simulink model "EngBrk_ExhFlpCtl"  (R2016b)
settings: configuration reference "CodeGenConfigSet" (kept outside this file)
values from neighbouring files (symbols this model uses):
  EngBrk_pExhFlpBstDflVal_C = Calibration.Parameter    [init_EngBrk_ExhFlpCtl.m]
  EngBrk_pExhFlpBstOn_C = Calibration.Parameter    [init_EngBrk_ExhFlpCtl.m]
  EngBrk_rExhFlpBrkLvl_C = Calibration.Parameter    [init_EngBrk_ExhFlpCtl.m]
  EngBrk_tiExhFlpBstOn_C = Calibration.Parameter    [init_EngBrk_ExhFlpCtl.m]
  PRC_ZERO = uint8(0)    [init_EngBrk_ExhFlpCtl.m]
undefined symbols (not defined in the file or in its folder): EngBrk_ExhFlpCtl_DT
settings Model: Creator=lenovo  LastModifiedBy=lenovo
settings ConfigSetRef: SourceLocation=Base Workspace

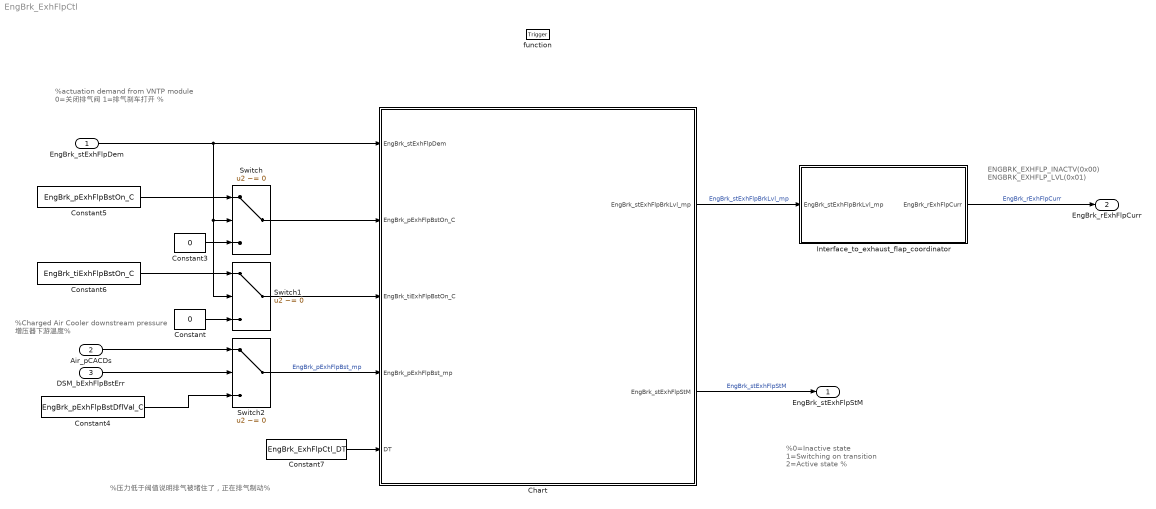
== system EngBrk_ExhFlpCtl ==
  note: %actuation demand from VNTP module
      | 0=关闭排气阀
      | 1=排气刹车打开 %
  note: ENGBRK_EXHFLP_INACTV(0x00)
      | ENGBRK_EXHFLP_LVL(0x01)
  note: %0=Inactive state
      | 1=Switching on transition
      | 2=Active state %
  note: %Charged Air Cooler downstream pressure
      | 增压器下游温度%
  note: %压力低于阀值说明排气被堵住了，正在排气制动%
  EngBrk_stExhFlpDem : Inport  Description=Activation demand to exhaust flap  OutMin=0  OutMax=1  OutDataTypeStr=boolean
  Air_pCACDs : Inport  Tag=kPa  Description=Air pressure downstream of the charge air cooler  Port=2  OutMin=-3276.8  OutMax=3276.7  OutDataTypeStr=AirPressure_kPa
  DSM_bExhFlpBstErr : Inport  Description=state of FId_ExhFlpBstErr  Port=3  OutMin=0  OutMax=1  OutDataTypeStr=boolean
  function : TriggerPort  TriggerType=function-call  VariantControl=Variant
  Chart : Stateflow chart  TreatAsAtomicUnit=on
  Constant : Constant  Value=0  OutDataTypeStr=Inherit: Inherit via back propagation
  Constant3 : Constant  Value=0  OutDataTypeStr=Inherit: Inherit via back propagation
  Constant4 : Constant  Value=EngBrk_pExhFlpBstDflVal_C
  Constant5 : Constant  Value=EngBrk_pExhFlpBstOn_C
  Constant6 : Constant  Value=EngBrk_tiExhFlpBstOn_C
  Constant7 : Constant  Value=EngBrk_ExhFlpCtl_DT  OutDataTypeStr=Inherit: Inherit via back propagation
  Interface_to_exhaust_flap_coordinator : Subsystem
  Switch : Switch  Criteria=u2 ~= 0  SaturateOnIntegerOverflow=on  InputSameDT=on
  Switch1 : Switch  Criteria=u2 ~= 0  SaturateOnIntegerOverflow=on  InputSameDT=on
  Switch2 : Switch  Criteria=u2 ~= 0  SaturateOnIntegerOverflow=on  InputSameDT=on
  EngBrk_stExhFlpStM : Outport  Description=Current status of the state machine in exhaust flap control  OutMin=0  OutMax=255  OutDataTypeStr=State_uint8
  EngBrk_rExhFlpCurr : Outport  Tag=%  Description=Actual status (process signal) of exhaust flap  Port=2  OutMin=-200  OutMax=200  OutDataTypeStr=DutyCycle_rate
  wires:
  Constant7/1 -> Chart/5(DT)
  Switch1/1 -> Chart/3(EngBrk_tiExhFlpBstOn_C)
  DSM_bExhFlpBstErr/1 -> Switch2/2
  EngBrk_stExhFlpDem/1 -> Switch/2, Switch1/2, Chart/1(EngBrk_stExhFlpDem)
  Chart/1(EngBrk_stExhFlpBrkLvl_mp) -> Interface_to_exhaust_flap_coordinator/1(EngBrk_stExhFlpBrkLvl_mp)  "EngBrk_stExhFlpBrkLvl_mp"
  Constant3/1 -> Switch/3
  Constant4/1 -> Switch2/3
  Air_pCACDs/1 -> Switch2/1
  Chart/2(EngBrk_stExhFlpStM) -> EngBrk_stExhFlpStM/1  "EngBrk_stExhFlpStM"
  Constant/1 -> Switch1/3
  Switch2/1 -> Chart/4(EngBrk_pExhFlpBst_mp)  "EngBrk_pExhFlpBst_mp"
  Switch/1 -> Chart/2(EngBrk_pExhFlpBstOn_C)
  Constant5/1 -> Switch/1
  Constant6/1 -> Switch1/1
  Interface_to_exhaust_flap_coordinator/1(EngBrk_rExhFlpCurr) -> EngBrk_rExhFlpCurr/1  "EngBrk_rExhFlpCurr"

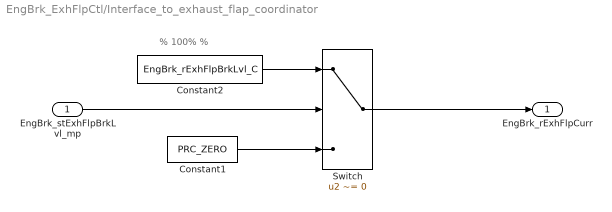
== system EngBrk_ExhFlpCtl/Interface_to_exhaust_flap_coordinator ==
  note: % 100% %
  EngBrk_stExhFlpBrkLvl_mp : Inport
  Constant1 : Constant  Value=PRC_ZERO  OutDataTypeStr=Inherit: Inherit via back propagation
  Constant2 : Constant  Value=EngBrk_rExhFlpBrkLvl_C
  Switch : Switch  Criteria=u2 ~= 0  SaturateOnIntegerOverflow=on  InputSameDT=on
  EngBrk_rExhFlpCurr : Outport
  wires:
  Switch/1 -> EngBrk_rExhFlpCurr/1
  Constant2/1 -> Switch/1
  EngBrk_stExhFlpBrkLvl_mp/1 -> Switch/2
  Constant1/1 -> Switch/3

== stateflow chart EngBrk_ExhFlpCtl/Chart ==
  state EXHFLP_WAIT_ON_REQ
    during:EngBrk_stExhFlpStM = 0;
    EngBrk_stExhFlpBrkLvl_mp = 0;
    timeout = 0;
  state EXHFLP_WAIT_SHUOFF_REQ
    during:EngBrk_stExhFlpStM = 2;
    EngBrk_stExhFlpBrkLvl_mp = 1;
  state EXHFLP_WAIT_BSTON_OR_TO
    during:EngBrk_stExhFlpStM = 1;
    EngBrk_stExhFlpBrkLvl_mp = 0;
    timeout = timeout + DT;
  (default) -> EXHFLP_WAIT_ON_REQ
  EXHFLP_WAIT_SHUOFF_REQ -> EXHFLP_WAIT_ON_REQ : [EngBrk_stExhFlpDem == 0 ]
  EXHFLP_WAIT_ON_REQ -> EXHFLP_WAIT_BSTON_OR_TO : [EngBrk_stExhFlpDem == 1]
  EXHFLP_WAIT_BSTON_OR_TO -> EXHFLP_WAIT_ON_REQ [order 1] : [EngBrk_stExhFlpDem == 0]
  EXHFLP_WAIT_BSTON_OR_TO -> EXHFLP_WAIT_SHUOFF_REQ [order 2] : [EngBrk_pExhFlpBst_mp <= EngBrk_pExhFlpBstOn_C...
      | || timeout >= EngBrk_tiExhFlpBstOn_C]
  data: EngBrk_stExhFlpBrkLvl_mp output; EngBrk_stExhFlpStM output; EngBrk_stExhFlpDem input; EngBrk_pExhFlpBstOn_C input; EngBrk_tiExhFlpBstOn_C input; EngBrk_pExhFlpBst_mp input; timeout local uint16; DT input
